simulink model "Compensadores_RLC_Paralelo"  (R2017a)
settings: Solver=VariableStepAuto  StartTime=0.0  StopTime=10.0  RelTol=1e-3
values from neighbouring files (symbols this model uses):
  C1 = 0.22    [Compensador_Adelanto.m]    (also in Compensador_Atraso.m = 0.0001)
  C2 = 0.010    (= 0.01)    [Compensador_Adelanto.m]    (also in Compensador_Atraso.m = 0.002)
  R1 = 3900    [Compensador_Adelanto.m]    (also in Compensador_Atraso.m = 2200)
  R2 = 1800    [Compensador_Adelanto.m]    (also in Compensador_Atraso.m = 3300)
  R3 = 2700    [Compensador_Adelanto.m]    (also in Compensador_Atraso.m = 1500)
  R4 = 4700    [Compensador_Adelanto.m]    (also in Compensador_Atraso.m)
libraries: fl_lib x7, nesl_utility x3
settings Model: Creator=Henry Alberto  LastModifiedBy=Henry Alberto

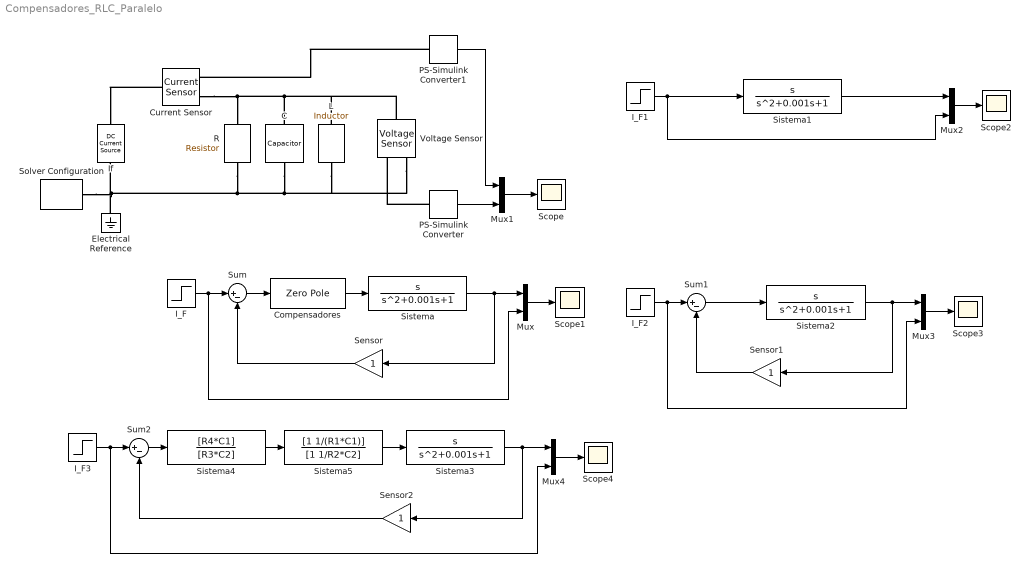
== system Compensadores_RLC_Paralelo ==
  C : fl_lib/Electrical/Electrical Elements/Capacitor  c=1 F  r=0 Ohm  g=0 1/Ohm  i_specify=off  i_priority=None  i=0 A  i_nominal_specify=off  i_nominal_unit=A  i_nominal_value=1  v_specify=off  v_priority=None  v=0 V  v_nominal_specify=off  v_nominal_unit=V  v_nominal_value=1  vc_specify=off  vc_priority=High  vc=0 V  vc_nominal_specify=off  vc_nominal_unit=V  vc_nominal_value=1
  Compensadores : ZeroPole  Poles=[1 -1]
  Current Sensor : fl_lib/Electrical/Electrical Sensors/Current Sensor
  Electrical Reference : fl_lib/Electrical/Electrical Elements/Electrical Reference
  I_F{,1..3} (4 alike) : Step  SampleTime=0
  If : fl_lib/Electrical/Electrical Sources/DC Current Source  i0=1 A
      settings: SourceProductName=Simscape  SourceProductBaseCode=SS
  L : fl_lib/Electrical/Electrical Elements/Inductor  l=1 H  r=0 Ohm  g=0 1/Ohm  i_specify=off  i_priority=None  i=0 A  i_nominal_specify=off  i_nominal_unit=A  i_nominal_value=1  v_specify=off  v_priority=None  v=0 V  v_nominal_specify=off  v_nominal_unit=V  v_nominal_value=1  i_L_specify=off  i_L_priority=High  i_L=0 A  i_L_nominal_specify=off  i_L_nominal_unit=A  i_L_nominal_value=1
  Mux{,1..4} (5 alike) : Mux  Inputs=2
  PS-Simulink Converter : nesl_utility/PS-Simulink Converter  PhysicalDomain=network_engine_domain  SubClassName=ps_output  LeftPortType=input  RightPortType=output  PseudoPeriodic=off  Frequencies=[]  Unit=1  AffineConversion=off
  PS-Simulink Converter1 : nesl_utility/PS-Simulink Converter  PhysicalDomain=network_engine_domain  SubClassName=ps_output  LeftPortType=input  RightPortType=output  PseudoPeriodic=off  Frequencies=[]  Unit=1  AffineConversion=off
  R : fl_lib/Electrical/Electrical Elements/Resistor  R=1000 Ohm  i_specify=off  i_priority=None  i=0 A  i_nominal_specify=off  i_nominal_unit=A  i_nominal_value=1  v_specify=off  v_priority=None  v=0 V  v_nominal_specify=off  v_nominal_unit=V  v_nominal_value=1
  Scope{,1..4} (5 alike) : Scope
  Sensor : Gain
  Sensor1 : Gain
  Sensor2 : Gain
  Sistema{,1..3} (4 alike) : TransferFcn  Numerator=[1 0]  Denominator=[1 0.001 1]
  Sistema4 : TransferFcn  Numerator=[R4*C1]  Denominator=[R3*C2]
  Sistema5 : TransferFcn  Numerator=[1 1/(R1*C1)]  Denominator=[1 1/R2*C2]
  Solver Configuration : nesl_utility/Solver Configuration  PhysicalDomain=network_engine_domain  SubClassName=solver  LeftPortType=input  RightPortType=generic  Accelerate=off  Tones=[]  Harmonics=[]  SimulateNoise=off  Profile=off  UseLocalSampling=off  EnableSwitchedLinearOptims=on  FrequencyDomain=off  UseCCode=off  RelTol=0.001  AbsTol=1e-06  MinStep=1e-09  ToWorkspace=off  RevertToSquareIcSolve=off  NumHomotopyIterations=100  PhasorMode=off  PhasorModeNumHarmonics=1  OverrideAbsTol=off  DoDC=off  ResidualTolerance=1e-09  UseLocalSolver=off  LocalSolverChoice=NE_BACKWARD_EULER_ADVANCER  LocalSolverSampleTime=0.001  DoFixedCost=off  MaxNonlinIter=3  MaxModeIter=2  LinearAlgebra=Sparse  DelaysMemoryBudget=1024  AutomaticFiltering=on  FilteringTimeConstant=0.001
  Sum : Sum  Inputs=|+-
  Sum1 : Sum  Inputs=|+-
  Sum2 : Sum  Inputs=|+-
  Voltage Sensor : fl_lib/Electrical/Electrical Sensors/Voltage Sensor
  wires:
  Mux/1 -> Scope1/1
  PS-Simulink Converter/1 -> Mux1/2
  Mux1/1 -> Scope/1
  PS-Simulink Converter1/1 -> Mux1/1
  I_F/1 -> Mux/2, Sum/1
  Sistema/1 -> Sensor/1, Mux/1
  Sensor/1 -> Sum/2
  Sistema1/1 -> Mux2/1
  Mux2/1 -> Scope2/1
  I_F1/1 -> Sistema1/1, Mux2/2
  Sum/1 -> Compensadores/1
  Compensadores/1 -> Sistema/1
  Sistema2/1 -> Sensor1/1, Mux3/1
  Mux3/1 -> Scope3/1
  Sum1/1 -> Sistema2/1
  Sensor1/1 -> Sum1/2
  I_F2/1 -> Mux3/2, Sum1/1
  Sistema3/1 -> Sensor2/1, Mux4/1
  Mux4/1 -> Scope4/1
  Sistema5/1 -> Sistema3/1
  Sum2/1 -> Sistema4/1
  Sensor2/1 -> Sum2/2
  I_F3/1 -> Mux4/2, Sum2/1
  Sistema4/1 -> Sistema5/1
  connections:
  C/LConn1 -- Voltage Sensor/LConn1 -- L/LConn1 -- R/LConn1 -- Current Sensor/RConn2
  R/RConn1 -- Voltage Sensor/RConn2 -- L/RConn1 -- C/RConn1 -- Electrical Reference/LConn1 -- Solver Configuration/RConn1 -- If/RConn1
  PS-Simulink Converter/LConn1 -- Voltage Sensor/RConn1
  Current Sensor/LConn1 -- If/LConn1
  PS-Simulink Converter1/LConn1 -- Current Sensor/RConn1
